simulink model "Plant"  (R2019a)
settings: Solver=VariableStepAuto  StartTime=0.0  StopTime=10.0  RelTol=1e-3
settings Model: Creator=AMIN  LastModifiedBy=AMIN
settings DataIOCC: SaveFormat=Array  ReturnWorkspaceOutputs=off

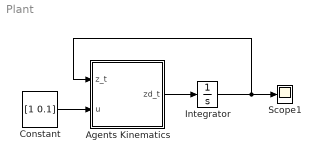
== system Plant ==
  Agents Kinematics : MATLAB Function  TreatAsAtomicUnit=on
  Constant : Constant  Value=[1 0.1]  VectorParams1D=off  OutDataTypeStr=Inherit: Inherit via back propagation
  Integrator : Integrator
  Scope1 : Scope
  wires:
  Constant/1 -> Agents Kinematics/2(u)
  Agents Kinematics/1(zd_t) -> Integrator/1
  Integrator/1 -> Agents Kinematics/1(z_t), Scope1/1

== matlab function Plant/Agents Kinematics ==
  data: z_t input; zd_t output; u input
function zd_t  = KIN(z_t,u)

n = size(u,1);
zd_t =zeros(n,3);

   for i=1:1:n
        
        [zd_t(i,1:2),zd_t(i,3)] = Agent_Kinematics(z_t(i,3),u(i,:));
        
    end 

end
